simulink model "Loopshaping_usingknob"  (R2023b)
settings: Solver=VariableStepAuto  StartTime=0.0  StopTime=50.0  RelTol=1e-3
settings Model: Creator=ADMIN  LastModifiedBy=ADMIN

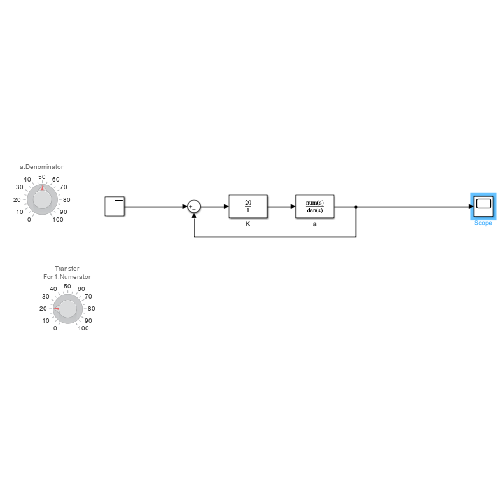
[thumbnail: Simulink's stored preview of the top-level diagram]
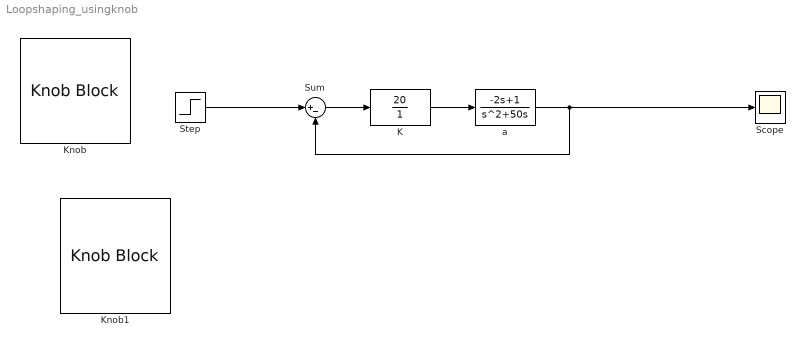
== system Loopshaping_usingknob ==
  K : TransferFcn  Numerator=20  Denominator=[1]
  Knob : KnobBlock
  Knob1 : KnobBlock
  Scope : Scope
  Step : Step  SampleTime=0
  Sum : Sum  Inputs=|+-
  a : TransferFcn  Numerator=[-2 1]  Denominator=[1,50,0]
  wires:
  Step/1 -> Sum/1
  a/1 -> Sum/2, Scope/1
  Sum/1 -> K/1
  K/1 -> a/1
